simulink model "quarter car model"  (R2026a)
settings: Solver=VariableStepAuto
settings Model: Creator=eonra  LastModifiedBy=eonra

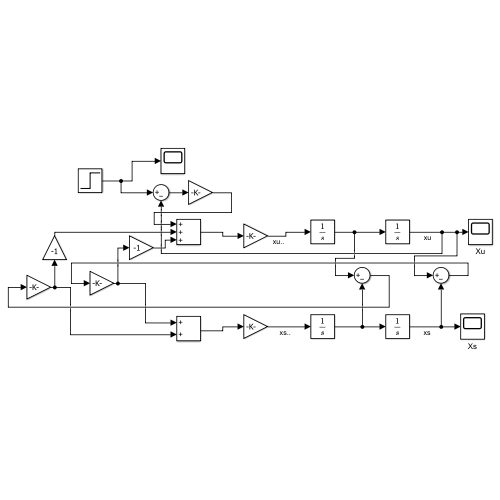
[thumbnail: Simulink's stored preview of the top-level diagram]
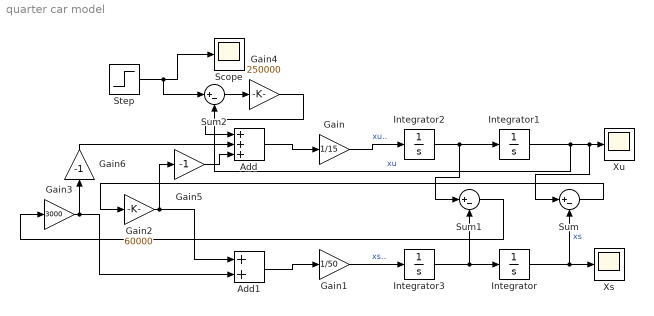
== system quarter car model ==
  Add : Sum  Inputs=+++
  Add1 : Sum
  Gain : Gain  Gain=1/15
  Gain1 : Gain  Gain=1/50
  Gain2 : Gain  Gain=60000
  Gain3 : Gain  Gain=3000
  Gain4 : Gain  Gain=250000
  Gain5 : Gain  Gain=-1
  Gain6 : Gain  Gain=-1
  Integrator{,1..3} (4 alike) : Integrator
  Scope : Scope
      settings: ActiveDisplayYMinimum=-1  ActiveDisplayYMaximum=1  DataLoggingVariableName=ScopeData2
  Step : Step  SampleTime=0
  Sum : Sum  Inputs=|+-
  Sum1 : Sum  Inputs=|+-
  Sum2 : Sum  Inputs=|+-
  Xs : Scope
      settings: ActiveDisplayYMinimum=-0.0882781623197395  ActiveDisplayYMaximum=1.5596942645661311
  Xu : Scope
      settings: ActiveDisplayYMinimum=-0.22872052241547425  ActiveDisplayYMaximum=1.821839960880435
  wires:
  Integrator1/1 -> Sum2/2, Sum/1, Xu/1  "xu"
  Integrator2/1 -> Sum1/1, Integrator1/1
  Integrator/1 -> Xs/1, Sum/2  "xs"
  Integrator3/1 -> Sum1/2, Integrator/1
  Gain/1 -> Integrator2/1  "xu.."
  Gain1/1 -> Integrator3/1  "xs.."
  Sum/1 -> Gain2/1
  Gain2/1 -> Add1/1, Gain5/1
  Sum1/1 -> Gain3/1
  Gain3/1 -> Add1/2, Gain6/1
  Add1/1 -> Gain1/1
  Step/1 -> Sum2/1, Scope/1
  Sum2/1 -> Gain4/1
  Gain4/1 -> Add/1
  Add/1 -> Gain/1
  Gain6/1 -> Add/2
  Gain5/1 -> Add/3
